simulink model "ApproachTargeting"  (R2014b)
settings: Solver=ode45  StartTime=0.0  StopTime=10.0  RelTol=1e-3
libraries: simulink x4
settings Model: Creator=Mark Agbayani  LastModifiedBy=Mark Agbayani

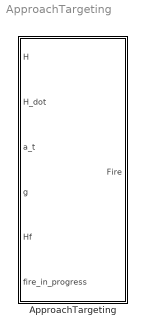
== system ApproachTargeting ==
  ApproachTargeting : Subsystem

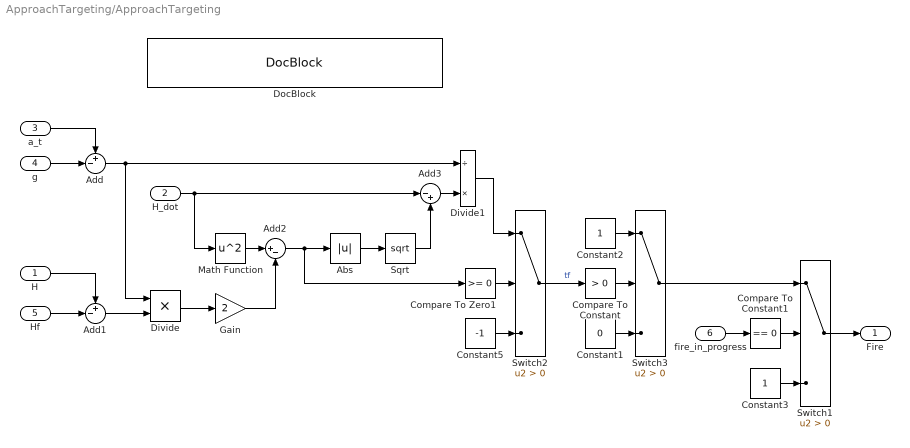
== system ApproachTargeting/ApproachTargeting ==
  H : Inport
  H_dot : Inport  Port=2
  a_t : Inport  Port=3
  g : Inport  Port=4
  Hf : Inport  Port=5
  fire_in_progress : Inport  Port=6
  Abs : Abs
  Add : Sum  Inputs=+-|
  Add1 : Sum  Inputs=+-|
  Add2 : Sum  Inputs=|+-
  Add3 : Sum  Inputs=|-+
  Compare To Constant : simulink/Logic and Bit Operations/Compare To Constant  relop=>  const=0  OutDataTypeStr=boolean
  Compare To Constant1 : simulink/Logic and Bit Operations/Compare To Constant  relop===  const=0  OutDataTypeStr=boolean
  Compare To Zero1 : simulink/Logic and Bit Operations/Compare To Zero  relop=>=  OutDataTypeStr=boolean
  Constant1 : Constant  Value=0
  Constant2 : Constant
  Constant3 : Constant
  Constant5 : Constant  Value=-1
  Divide : Product  Inputs=**
  Divide1 : Product  Inputs=/*
  DocBlock : simulink/Model-Wide Utilities/DocBlock  DocumentType=Text
      content=|
      | function Fire = ApproachTargeting(H,Hdot,a_t,g,Hf,fire_in_progress)
      |
      | Hi = H;
      | Hdoti = Hdot;
      |
      | if fire_in_progress == 0
      |
      |     if (Hdoti^2 - 2*(a_t - g)*(Hi - Hf)) >= 0
      |        tf = (-Hdoti + sqrt(Hdoti^2 - 2*(a_t - g)*(Hi - Hf)))/(a_t - g);
      |     else
      |       tf = -1;
      |     end
      |
      |     if tf > 0;
      |         Fire = true;
      |     else
      |         Fire = false;
      |     end
      | else
      |     Fire = true;
      | end
  Gain : Gain  Gain=2
  Math Function : Math  Operator=square  SaturateOnIntegerOverflow=on
  Sqrt : Sqrt  SaturateOnIntegerOverflow=on
  Switch1 : Switch  Criteria=u2 > Threshold
  Switch2 : Switch  Criteria=u2 > Threshold
  Switch3 : Switch  Criteria=u2 > Threshold
  Fire : Outport  InitialOutput=[0 0 1]'
  wires:
  Switch1/1 -> Fire/1
  fire_in_progress/1 -> Compare To Constant1/1
  Compare To Constant1/1 -> Switch1/2
  Constant3/1 -> Switch1/3
  H_dot/1 -> Math Function/1, Add3/1
  a_t/1 -> Add/1
  g/1 -> Add/2
  Hf/1 -> Add1/2
  H/1 -> Add1/1
  Add/1 -> Divide/1, Divide1/1
  Add1/1 -> Divide/2
  Divide/1 -> Gain/1
  Add2/1 -> Compare To Zero1/1, Abs/1
  Math Function/1 -> Add2/1
  Gain/1 -> Add2/2
  Compare To Zero1/1 -> Switch2/2
  Abs/1 -> Sqrt/1
  Divide1/1 -> Switch2/1
  Constant5/1 -> Switch2/3
  Switch2/1 -> Compare To Constant/1  "tf"
  Compare To Constant/1 -> Switch3/2
  Constant1/1 -> Switch3/3
  Switch3/1 -> Switch1/1
  Add3/1 -> Divide1/2
  Sqrt/1 -> Add3/2
  Constant2/1 -> Switch3/1
